simulink model "ASM_Traffic_V2X_Complete_Model_2"  (R2019a)
settings: Solver=ode1  StartTime=SIM.tstart.v  StopTime=Inf  FixedStep=SIM.StepSize.v  RelTol=1e-3
PostLoadFcn:
  | if any(exist('dsrtsu_mdlpostloadfcn', 'file') ~= 0), dsrtsu_mdlpostloadfcn('Execute', bdroot); end
  | try, asm_mdl_postloadfcn(bdroot, 'UpdateModel', 2200); catch, disp(lasterr); end,
undefined symbols (not defined in the file): _SensorPnts_1, _SensorPnts_13, _SensorPnts_17, _SensorPnts_21, _SensorPnts_25, _SensorPnts_29, _SensorPnts_33, _SensorPnts_37, _SensorPnts_41, _SensorPnts_45, _SensorPnts_49, _SensorPnts_5, _SensorPnts_53, _SensorPnts_57, _SensorPnts_9, _to_, CPT, G5A, ITS, MDL, rad, s_to_rpm, SIM
libraries: simulink x169, ASM_VehicleDynamics_lib x126, ASM_Traffic_lib x83, ASM_Utils_lib x49, mdbs x45, ASM_Environment_lib x17, dspindex x12, dsaV2xLibraryAux x10, dsmpblib x6, dsaV2xAsn1Library x4, dsaV2xLibrary x4, ASM_BrakeHydraulics_lib x4
(part 25 of 36)

== system ASM_Traffic_V2X_Complete_Model_2/MDL/Environment/Traffic/Sensors/Object_Sensor_2D/SensorParameters ==
  Demux{,1..6} (7 alike) : Demux  Outputs=3
  Mux{1..7} (7 alike) : Mux  Inputs=14
  OBJECT_SENSOR_2D_PARAMETERS_1 : ASM_Traffic_lib/Sensors/Object_Sensor_2D/OBJECT_SENSOR_2D_PARAMETERS  Tag=ASM_SUBCOMPONENT  Sw_Sensor_Enable=MDL.Traffic.Sensors.ObjectSensor2D_1.Sw_Sensor_Enable  Const_SensorIdx=MDL.Traffic.Sensors.ObjectSensor2D_1.Const_SensorIdx  Const_t_Offs_Sensor=MDL.Traffic.Sensors.ObjectSensor2D_1.Const_t_Offs_Sensor  Const_t_Cycle_Sensor=MDL.Traffic.Sensors.ObjectSensor2D_1.Const_t_Cycle_Sensor  Const_t_Delay_SensorOutput=MDL.Traffic.Sensors.ObjectSensor2D_1.Const_t_Delay_SensorOutput  Const_Pos_Sensor_Apex_CoorSys_V=MDL.Traffic.Sensors.ObjectSensor2D_1.Const_Pos_Sensor_Apex_CoorSys_V  Const_Angle_z_Orientation_Sensor_CoorSys_V=MDL.Traffic.Sensors.ObjectSensor2D_1.Const_Angle_z_Orientation_Sensor_CoorSys_V  Const_Angle_ScopeZone_Horizontal=MDL.Traffic.Sensors.ObjectSensor2D_1.Const_Angle_ScopeZone_Horizontal  Const_Length_ScopeZone=MDL.Traffic.Sensors.ObjectSensor2D_1.Const_Length_ScopeZone  Const_Num_SensorRays_Used=MDL.Traffic.Sensors.ObjectSensor2D_1.Const_Num_SensorRays_Used  Sw_Sensor_Detection_Mode=MDL.Traffic.Sensors.ObjectSensor2D_1.Sw_Sensor_Detection_Mode  Sw_Object_Detection_Mode=MDL.Traffic.Sensors.ObjectSensor2D_1.Sw_Object_Detection_Mode  ASMProperties=struct('Name','OBJECT_SENSOR_2D_PARAMETERS','Version','5.0','Library','ASM_Traffic_lib')  ASMInstanceName=object_sensor_2d_parameters  ASMInstanceID=1
  OBJECT_SENSOR_2D_PARAMETERS_2 : ASM_Traffic_lib/Sensors/Object_Sensor_2D/OBJECT_SENSOR_2D_PARAMETERS  Tag=ASM_SUBCOMPONENT  Sw_Sensor_Enable=MDL.Traffic.Sensors.ObjectSensor2D_2.Sw_Sensor_Enable  Const_SensorIdx=MDL.Traffic.Sensors.ObjectSensor2D_2.Const_SensorIdx  Const_t_Offs_Sensor=MDL.Traffic.Sensors.ObjectSensor2D_2.Const_t_Offs_Sensor  Const_t_Cycle_Sensor=MDL.Traffic.Sensors.ObjectSensor2D_2.Const_t_Cycle_Sensor  Const_t_Delay_SensorOutput=MDL.Traffic.Sensors.ObjectSensor2D_2.Const_t_Delay_SensorOutput  Const_Pos_Sensor_Apex_CoorSys_V=MDL.Traffic.Sensors.ObjectSensor2D_2.Const_Pos_Sensor_Apex_CoorSys_V  Const_Angle_z_Orientation_Sensor_CoorSys_V=MDL.Traffic.Sensors.ObjectSensor2D_2.Const_Angle_z_Orientation_Sensor_CoorSys_V  Const_Angle_ScopeZone_Horizontal=MDL.Traffic.Sensors.ObjectSensor2D_2.Const_Angle_ScopeZone_Horizontal  Const_Length_ScopeZone=MDL.Traffic.Sensors.ObjectSensor2D_2.Const_Length_ScopeZone  Const_Num_SensorRays_Used=MDL.Traffic.Sensors.ObjectSensor2D_2.Const_Num_SensorRays_Used  Sw_Sensor_Detection_Mode=MDL.Traffic.Sensors.ObjectSensor2D_2.Sw_Sensor_Detection_Mode  Sw_Object_Detection_Mode=MDL.Traffic.Sensors.ObjectSensor2D_2.Sw_Object_Detection_Mode  ASMProperties=struct('Name','OBJECT_SENSOR_2D_PARAMETERS','Version','5.0','Library','ASM_Traffic_lib')  ASMInstanceName=object_sensor_2d_parameters  ASMInstanceID=2
      settings: AttributesFormatString=Instance Name: object_sensor_2d_parameters\nInstance ID: 2
  OBJECT_SENSOR_2D_PARAMETERS_3 : ASM_Traffic_lib/Sensors/Object_Sensor_2D/OBJECT_SENSOR_2D_PARAMETERS  Tag=ASM_SUBCOMPONENT  Sw_Sensor_Enable=MDL.Traffic.Sensors.ObjectSensor2D_3.Sw_Sensor_Enable  Const_SensorIdx=MDL.Traffic.Sensors.ObjectSensor2D_3.Const_SensorIdx  Const_t_Offs_Sensor=MDL.Traffic.Sensors.ObjectSensor2D_3.Const_t_Offs_Sensor  Const_t_Cycle_Sensor=MDL.Traffic.Sensors.ObjectSensor2D_3.Const_t_Cycle_Sensor  Const_t_Delay_SensorOutput=MDL.Traffic.Sensors.ObjectSensor2D_3.Const_t_Delay_SensorOutput  Const_Pos_Sensor_Apex_CoorSys_V=MDL.Traffic.Sensors.ObjectSensor2D_3.Const_Pos_Sensor_Apex_CoorSys_V  Const_Angle_z_Orientation_Sensor_CoorSys_V=MDL.Traffic.Sensors.ObjectSensor2D_3.Const_Angle_z_Orientation_Sensor_CoorSys_V  Const_Angle_ScopeZone_Horizontal=MDL.Traffic.Sensors.ObjectSensor2D_3.Const_Angle_ScopeZone_Horizontal  Const_Length_ScopeZone=MDL.Traffic.Sensors.ObjectSensor2D_3.Const_Length_ScopeZone  Const_Num_SensorRays_Used=MDL.Traffic.Sensors.ObjectSensor2D_3.Const_Num_SensorRays_Used  Sw_Sensor_Detection_Mode=MDL.Traffic.Sensors.ObjectSensor2D_3.Sw_Sensor_Detection_Mode  Sw_Object_Detection_Mode=MDL.Traffic.Sensors.ObjectSensor2D_3.Sw_Object_Detection_Mode  ASMProperties=struct('Name','OBJECT_SENSOR_2D_PARAMETERS','Version','5.0','Library','ASM_Traffic_lib')  ASMInstanceName=object_sensor_2d_parameters  ASMInstanceID=3
      settings: AttributesFormatString=Instance Name: object_sensor_2d_parameters\nInstance ID: 3
  OBJECT_SENSOR_2D_PARAMETERS_4 : ASM_Traffic_lib/Sensors/Object_Sensor_2D/OBJECT_SENSOR_2D_PARAMETERS  Tag=ASM_SUBCOMPONENT  Sw_Sensor_Enable=MDL.Traffic.Sensors.ObjectSensor2D_4.Sw_Sensor_Enable  Const_SensorIdx=MDL.Traffic.Sensors.ObjectSensor2D_4.Const_SensorIdx  Const_t_Offs_Sensor=MDL.Traffic.Sensors.ObjectSensor2D_4.Const_t_Offs_Sensor  Const_t_Cycle_Sensor=MDL.Traffic.Sensors.ObjectSensor2D_4.Const_t_Cycle_Sensor  Const_t_Delay_SensorOutput=MDL.Traffic.Sensors.ObjectSensor2D_4.Const_t_Delay_SensorOutput  Const_Pos_Sensor_Apex_CoorSys_V=MDL.Traffic.Sensors.ObjectSensor2D_4.Const_Pos_Sensor_Apex_CoorSys_V  Const_Angle_z_Orientation_Sensor_CoorSys_V=MDL.Traffic.Sensors.ObjectSensor2D_4.Const_Angle_z_Orientation_Sensor_CoorSys_V  Const_Angle_ScopeZone_Horizontal=MDL.Traffic.Sensors.ObjectSensor2D_4.Const_Angle_ScopeZone_Horizontal  Const_Length_ScopeZone=MDL.Traffic.Sensors.ObjectSensor2D_4.Const_Length_ScopeZone  Const_Num_SensorRays_Used=MDL.Traffic.Sensors.ObjectSensor2D_4.Const_Num_SensorRays_Used  Sw_Sensor_Detection_Mode=MDL.Traffic.Sensors.ObjectSensor2D_4.Sw_Sensor_Detection_Mode  Sw_Object_Detection_Mode=MDL.Traffic.Sensors.ObjectSensor2D_4.Sw_Object_Detection_Mode  ASMProperties=struct('Name','OBJECT_SENSOR_2D_PARAMETERS','Version','5.0','Library','ASM_Traffic_lib')  ASMInstanceName=object_sensor_2d_parameters  ASMInstanceID=4
      settings: AttributesFormatString=Instance Name: object_sensor_2d_parameters\nInstance ID: 4
  OBJECT_SENSOR_2D_PARAMETERS_5 : ASM_Traffic_lib/Sensors/Object_Sensor_2D/OBJECT_SENSOR_2D_PARAMETERS  Tag=ASM_SUBCOMPONENT  Sw_Sensor_Enable=MDL.Traffic.Sensors.ObjectSensor2D_5.Sw_Sensor_Enable  Const_SensorIdx=MDL.Traffic.Sensors.ObjectSensor2D_5.Const_SensorIdx  Const_t_Offs_Sensor=MDL.Traffic.Sensors.ObjectSensor2D_5.Const_t_Offs_Sensor  Const_t_Cycle_Sensor=MDL.Traffic.Sensors.ObjectSensor2D_5.Const_t_Cycle_Sensor  Const_t_Delay_SensorOutput=MDL.Traffic.Sensors.ObjectSensor2D_5.Const_t_Delay_SensorOutput  Const_Pos_Sensor_Apex_CoorSys_V=MDL.Traffic.Sensors.ObjectSensor2D_5.Const_Pos_Sensor_Apex_CoorSys_V  Const_Angle_z_Orientation_Sensor_CoorSys_V=MDL.Traffic.Sensors.ObjectSensor2D_5.Const_Angle_z_Orientation_Sensor_CoorSys_V  Const_Angle_ScopeZone_Horizontal=MDL.Traffic.Sensors.ObjectSensor2D_5.Const_Angle_ScopeZone_Horizontal  Const_Length_ScopeZone=MDL.Traffic.Sensors.ObjectSensor2D_5.Const_Length_ScopeZone  Const_Num_SensorRays_Used=MDL.Traffic.Sensors.ObjectSensor2D_5.Const_Num_SensorRays_Used  Sw_Sensor_Detection_Mode=MDL.Traffic.Sensors.ObjectSensor2D_5.Sw_Sensor_Detection_Mode  Sw_Object_Detection_Mode=MDL.Traffic.Sensors.ObjectSensor2D_5.Sw_Object_Detection_Mode  ASMProperties=struct('Name','OBJECT_SENSOR_2D_PARAMETERS','Version','5.0','Library','ASM_Traffic_lib')  ASMInstanceName=object_sensor_2d_parameters  ASMInstanceID=5
      settings: AttributesFormatString=Instance Name: object_sensor_2d_parameters\nInstance ID: 5
  OBJECT_SENSOR_2D_PARAMETERS_6 : ASM_Traffic_lib/Sensors/Object_Sensor_2D/OBJECT_SENSOR_2D_PARAMETERS  Tag=ASM_SUBCOMPONENT  Sw_Sensor_Enable=MDL.Traffic.Sensors.ObjectSensor2D_6.Sw_Sensor_Enable  Const_SensorIdx=MDL.Traffic.Sensors.ObjectSensor2D_6.Const_SensorIdx  Const_t_Offs_Sensor=MDL.Traffic.Sensors.ObjectSensor2D_6.Const_t_Offs_Sensor  Const_t_Cycle_Sensor=MDL.Traffic.Sensors.ObjectSensor2D_6.Const_t_Cycle_Sensor  Const_t_Delay_SensorOutput=MDL.Traffic.Sensors.ObjectSensor2D_6.Const_t_Delay_SensorOutput  Const_Pos_Sensor_Apex_CoorSys_V=MDL.Traffic.Sensors.ObjectSensor2D_6.Const_Pos_Sensor_Apex_CoorSys_V  Const_Angle_z_Orientation_Sensor_CoorSys_V=MDL.Traffic.Sensors.ObjectSensor2D_6.Const_Angle_z_Orientation_Sensor_CoorSys_V  Const_Angle_ScopeZone_Horizontal=MDL.Traffic.Sensors.ObjectSensor2D_6.Const_Angle_ScopeZone_Horizontal  Const_Length_ScopeZone=MDL.Traffic.Sensors.ObjectSensor2D_6.Const_Length_ScopeZone  Const_Num_SensorRays_Used=MDL.Traffic.Sensors.ObjectSensor2D_6.Const_Num_SensorRays_Used  Sw_Sensor_Detection_Mode=MDL.Traffic.Sensors.ObjectSensor2D_6.Sw_Sensor_Detection_Mode  Sw_Object_Detection_Mode=MDL.Traffic.Sensors.ObjectSensor2D_6.Sw_Object_Detection_Mode  ASMProperties=struct('Name','OBJECT_SENSOR_2D_PARAMETERS','Version','5.0','Library','ASM_Traffic_lib')  ASMInstanceName=object_sensor_2d_parameters  ASMInstanceID=6
      settings: AttributesFormatString=Instance Name: object_sensor_2d_parameters\nInstance ID: 6
  OBJECT_SENSOR_2D_PARAMETERS_7 : ASM_Traffic_lib/Sensors/Object_Sensor_2D/OBJECT_SENSOR_2D_PARAMETERS  Tag=ASM_SUBCOMPONENT  Sw_Sensor_Enable=MDL.Traffic.Sensors.ObjectSensor2D_7.Sw_Sensor_Enable  Const_SensorIdx=MDL.Traffic.Sensors.ObjectSensor2D_7.Const_SensorIdx  Const_t_Offs_Sensor=MDL.Traffic.Sensors.ObjectSensor2D_7.Const_t_Offs_Sensor  Const_t_Cycle_Sensor=MDL.Traffic.Sensors.ObjectSensor2D_7.Const_t_Cycle_Sensor  Const_t_Delay_SensorOutput=MDL.Traffic.Sensors.ObjectSensor2D_7.Const_t_Delay_SensorOutput  Const_Pos_Sensor_Apex_CoorSys_V=MDL.Traffic.Sensors.ObjectSensor2D_7.Const_Pos_Sensor_Apex_CoorSys_V  Const_Angle_z_Orientation_Sensor_CoorSys_V=MDL.Traffic.Sensors.ObjectSensor2D_7.Const_Angle_z_Orientation_Sensor_CoorSys_V  Const_Angle_ScopeZone_Horizontal=MDL.Traffic.Sensors.ObjectSensor2D_7.Const_Angle_ScopeZone_Horizontal  Const_Length_ScopeZone=MDL.Traffic.Sensors.ObjectSensor2D_7.Const_Length_ScopeZone  Const_Num_SensorRays_Used=MDL.Traffic.Sensors.ObjectSensor2D_7.Const_Num_SensorRays_Used  Sw_Sensor_Detection_Mode=MDL.Traffic.Sensors.ObjectSensor2D_7.Sw_Sensor_Detection_Mode  Sw_Object_Detection_Mode=MDL.Traffic.Sensors.ObjectSensor2D_7.Sw_Object_Detection_Mode  ASMProperties=struct('Name','OBJECT_SENSOR_2D_PARAMETERS','Version','5.0','Library','ASM_Traffic_lib')  ASMInstanceName=object_sensor_2d_parameters  ASMInstanceID=7
      settings: AttributesFormatString=Instance Name: object_sensor_2d_parameters\nInstance ID: 7
  Vector Concatenate : Concatenate  NumInputs=7  Mode=Multidimensional array  ConcatenateDimension=2
  Sensor_Data[] : Outport
  tag scope: ASMBUS_Environment_Traffic_2DObjSensor1_Parameter=global, ASMBUS_Environment_Traffic_2DObjSensor2_Parameter=global, ASMBUS_Environment_Traffic_2DObjSensor3_Parameter=global, ASMBUS_Environment_Traffic_2DObjSensor4_Parameter=global, ASMBUS_Environment_Traffic_2DObjSensor5_Parameter=global, ASMBUS_Environment_Traffic_2DObjSensor6_Parameter=global, ASMBUS_Environment_Traffic_2DObjSensor7_Parameter=global
  wires:
  OBJECT_SENSOR_2D_PARAMETERS_3/13 -> Mux3/14
  OBJECT_SENSOR_2D_PARAMETERS_4/13 -> Mux4/14
  OBJECT_SENSOR_2D_PARAMETERS_7/13 -> Mux7/14
  OBJECT_SENSOR_2D_PARAMETERS_6/13 -> Mux6/14
  OBJECT_SENSOR_2D_PARAMETERS_5/13 -> Mux5/14
  OBJECT_SENSOR_2D_PARAMETERS_2/13 -> Mux2/14
  OBJECT_SENSOR_2D_PARAMETERS_1/13 -> Mux1/14
  OBJECT_SENSOR_2D_PARAMETERS_7/12 -> Mux7/13
  OBJECT_SENSOR_2D_PARAMETERS_7/11 -> Mux7/12
  OBJECT_SENSOR_2D_PARAMETERS_7/10 -> Mux7/11
  OBJECT_SENSOR_2D_PARAMETERS_7/9 -> Mux7/10
  OBJECT_SENSOR_2D_PARAMETERS_7/8 -> Mux7/9
  OBJECT_SENSOR_2D_PARAMETERS_7/6 -> Mux7/5
  OBJECT_SENSOR_2D_PARAMETERS_7/5 -> Mux7/4
  OBJECT_SENSOR_2D_PARAMETERS_7/4 -> Mux7/3
  OBJECT_SENSOR_2D_PARAMETERS_7/3 -> Mux7/2
  OBJECT_SENSOR_2D_PARAMETERS_7/2 -> Mux7/1
  Demux6/3 -> Mux7/8
  Demux6/2 -> Mux7/7
  Demux6/1 -> Mux7/6
  Mux7/1 -> Vector Concatenate/7
  OBJECT_SENSOR_2D_PARAMETERS_7/7 -> Demux6/1
  OBJECT_SENSOR_2D_PARAMETERS_6/12 -> Mux6/13
  OBJECT_SENSOR_2D_PARAMETERS_6/11 -> Mux6/12
  OBJECT_SENSOR_2D_PARAMETERS_6/10 -> Mux6/11
  OBJECT_SENSOR_2D_PARAMETERS_6/9 -> Mux6/10
  OBJECT_SENSOR_2D_PARAMETERS_6/8 -> Mux6/9
  OBJECT_SENSOR_2D_PARAMETERS_6/6 -> Mux6/5
  OBJECT_SENSOR_2D_PARAMETERS_6/5 -> Mux6/4
  OBJECT_SENSOR_2D_PARAMETERS_6/4 -> Mux6/3
  OBJECT_SENSOR_2D_PARAMETERS_6/3 -> Mux6/2
  OBJECT_SENSOR_2D_PARAMETERS_6/2 -> Mux6/1
  Demux5/3 -> Mux6/8
  Demux5/2 -> Mux6/7
  Demux5/1 -> Mux6/6
  Mux6/1 -> Vector Concatenate/6
  OBJECT_SENSOR_2D_PARAMETERS_6/7 -> Demux5/1
  OBJECT_SENSOR_2D_PARAMETERS_5/12 -> Mux5/13
  OBJECT_SENSOR_2D_PARAMETERS_5/11 -> Mux5/12
  OBJECT_SENSOR_2D_PARAMETERS_5/10 -> Mux5/11
  OBJECT_SENSOR_2D_PARAMETERS_5/9 -> Mux5/10
  OBJECT_SENSOR_2D_PARAMETERS_5/8 -> Mux5/9
  OBJECT_SENSOR_2D_PARAMETERS_5/6 -> Mux5/5
  OBJECT_SENSOR_2D_PARAMETERS_5/5 -> Mux5/4
  OBJECT_SENSOR_2D_PARAMETERS_5/4 -> Mux5/3
  OBJECT_SENSOR_2D_PARAMETERS_5/3 -> Mux5/2
  OBJECT_SENSOR_2D_PARAMETERS_5/2 -> Mux5/1
  Demux4/3 -> Mux5/8
  Demux4/2 -> Mux5/7
  Demux4/1 -> Mux5/6
  Mux5/1 -> Vector Concatenate/5
  OBJECT_SENSOR_2D_PARAMETERS_5/7 -> Demux4/1
  OBJECT_SENSOR_2D_PARAMETERS_4/12 -> Mux4/13
  OBJECT_SENSOR_2D_PARAMETERS_4/11 -> Mux4/12
  OBJECT_SENSOR_2D_PARAMETERS_4/10 -> Mux4/11
  OBJECT_SENSOR_2D_PARAMETERS_4/9 -> Mux4/10
  OBJECT_SENSOR_2D_PARAMETERS_4/8 -> Mux4/9
  OBJECT_SENSOR_2D_PARAMETERS_4/6 -> Mux4/5
  OBJECT_SENSOR_2D_PARAMETERS_4/5 -> Mux4/4
  OBJECT_SENSOR_2D_PARAMETERS_4/4 -> Mux4/3
  OBJECT_SENSOR_2D_PARAMETERS_4/3 -> Mux4/2
  OBJECT_SENSOR_2D_PARAMETERS_4/2 -> Mux4/1
  Demux3/3 -> Mux4/8
  Demux3/2 -> Mux4/7
  Demux3/1 -> Mux4/6
  Mux4/1 -> Vector Concatenate/4
  OBJECT_SENSOR_2D_PARAMETERS_4/7 -> Demux3/1
  OBJECT_SENSOR_2D_PARAMETERS_7/1 -> [ASMBUS_Environment_Traffic_2DObjSensor7_Parameter]
  OBJECT_SENSOR_2D_PARAMETERS_6/1 -> [ASMBUS_Environment_Traffic_2DObjSensor6_Parameter]
  OBJECT_SENSOR_2D_PARAMETERS_5/1 -> [ASMBUS_Environment_Traffic_2DObjSensor5_Parameter]
  OBJECT_SENSOR_2D_PARAMETERS_4/1 -> [ASMBUS_Environment_Traffic_2DObjSensor4_Parameter]
  OBJECT_SENSOR_2D_PARAMETERS_3/12 -> Mux3/13
  OBJECT_SENSOR_2D_PARAMETERS_2/12 -> Mux2/13
  OBJECT_SENSOR_2D_PARAMETERS_1/12 -> Mux1/13
  OBJECT_SENSOR_2D_PARAMETERS_3/11 -> Mux3/12
  OBJECT_SENSOR_2D_PARAMETERS_3/10 -> Mux3/11
  OBJECT_SENSOR_2D_PARAMETERS_3/9 -> Mux3/10
  OBJECT_SENSOR_2D_PARAMETERS_3/8 -> Mux3/9
  OBJECT_SENSOR_2D_PARAMETERS_3/6 -> Mux3/5
  OBJECT_SENSOR_2D_PARAMETERS_3/5 -> Mux3/4
  OBJECT_SENSOR_2D_PARAMETERS_3/4 -> Mux3/3
  OBJECT_SENSOR_2D_PARAMETERS_3/3 -> Mux3/2
  OBJECT_SENSOR_2D_PARAMETERS_3/2 -> Mux3/1
  Demux2/3 -> Mux3/8
  Demux2/2 -> Mux3/7
  Demux2/1 -> Mux3/6
  Mux3/1 -> Vector Concatenate/3
  OBJECT_SENSOR_2D_PARAMETERS_3/7 -> Demux2/1
  OBJECT_SENSOR_2D_PARAMETERS_3/1 -> [ASMBUS_Environment_Traffic_2DObjSensor3_Parameter]
  OBJECT_SENSOR_2D_PARAMETERS_2/11 -> Mux2/12
  OBJECT_SENSOR_2D_PARAMETERS_2/10 -> Mux2/11
  OBJECT_SENSOR_2D_PARAMETERS_2/9 -> Mux2/10
  OBJECT_SENSOR_2D_PARAMETERS_2/8 -> Mux2/9
  OBJECT_SENSOR_2D_PARAMETERS_2/6 -> Mux2/5
  OBJECT_SENSOR_2D_PARAMETERS_2/5 -> Mux2/4
  OBJECT_SENSOR_2D_PARAMETERS_2/4 -> Mux2/3
  OBJECT_SENSOR_2D_PARAMETERS_2/3 -> Mux2/2
  OBJECT_SENSOR_2D_PARAMETERS_2/2 -> Mux2/1
  Demux1/3 -> Mux2/8
  Demux1/2 -> Mux2/7
  Demux1/1 -> Mux2/6
  Mux2/1 -> Vector Concatenate/2
  OBJECT_SENSOR_2D_PARAMETERS_2/7 -> Demux1/1
  OBJECT_SENSOR_2D_PARAMETERS_2/1 -> [ASMBUS_Environment_Traffic_2DObjSensor2_Parameter]
  OBJECT_SENSOR_2D_PARAMETERS_1/11 -> Mux1/12
  OBJECT_SENSOR_2D_PARAMETERS_1/10 -> Mux1/11
  OBJECT_SENSOR_2D_PARAMETERS_1/9 -> Mux1/10
  OBJECT_SENSOR_2D_PARAMETERS_1/8 -> Mux1/9
  OBJECT_SENSOR_2D_PARAMETERS_1/6 -> Mux1/5
  OBJECT_SENSOR_2D_PARAMETERS_1/5 -> Mux1/4
  OBJECT_SENSOR_2D_PARAMETERS_1/4 -> Mux1/3
  OBJECT_SENSOR_2D_PARAMETERS_1/3 -> Mux1/2
  OBJECT_SENSOR_2D_PARAMETERS_1/2 -> Mux1/1
  Demux/3 -> Mux1/8
  Demux/2 -> Mux1/7
  Demux/1 -> Mux1/6
  Vector Concatenate/1 -> Sensor_Data[]/1
  Mux1/1 -> Vector Concatenate/1
  OBJECT_SENSOR_2D_PARAMETERS_1/7 -> Demux/1
  OBJECT_SENSOR_2D_PARAMETERS_1/1 -> [ASMBUS_Environment_Traffic_2DObjSensor1_Parameter]

== system ASM_Traffic_V2X_Complete_Model_2/MDL/Environment/Traffic/Sensors/Object_Sensor_3D/ASMSignalCollector ==
  Bus Creator : BusCreator  Inputs=5
  Bus Creator1 : BusCreator  Inputs=6
  Bus Creator2 : BusCreator  Inputs=6
  Bus Creator3 : BusCreator  Inputs=6
  Bus Selector : BusSelector  OutputSignals=SensorIndex,Info,SensorOutput
  Bus Selector1 : BusSelector  OutputSignals=SensorIndex,Info,SensorOutput
  Bus Selector2 : BusSelector  OutputSignals=SensorIndex,Info,SensorOutput
  tag scope: ASMBUS_Environment_Trafffic_Sensors_Object_Sensor_3D=global
  wires:
  [ASMBUS_Environment_Traffic_3DObjSensor3_RadarEffects] -> Bus Creator3/5  "RadarEffects"
  [ASMBUS_Environment_Traffic_3DObjSensor3_CustomPoints] -> Bus Creator3/6  "CustomPoints"
  [ASMBUS_Environment_Traffic_3DObjSensor2_RadarEffects] -> Bus Creator2/5  "RadarEffects"
  [ASMBUS_Environment_Traffic_3DObjSensor2_CustomPoints] -> Bus Creator2/6  "CustomPoints"
  [ASMBUS_Environment_Traffic_3DObjSensor1_CustomPoints] -> Bus Creator1/6  "CustomPoints"
  [ASMBUS_Environment_Traffic_3DObjSensor1_RadarEffects] -> Bus Creator1/5  "RadarEffects"
  [ASMBUS_Environment_Traffic_SamplePulse] -> Bus Creator/1  "Sample_Pulse"
  [ASMBUS_Environment_Traffic_SensorScheduler] -> Bus Creator/2  "Sensor_Scheduler"
  Bus Selector/3 -> Bus Creator1/4  "<SensorOutput>"
  Bus Selector/2 -> Bus Creator1/3  "<Info>"
  Bus Selector2/3 -> Bus Creator3/4  "<SensorOutput>"
  Bus Selector2/2 -> Bus Creator3/3  "<Info>"
  Bus Selector1/3 -> Bus Creator2/4  "<SensorOutput>"
  Bus Selector1/2 -> Bus Creator2/3  "<Info>"
  Bus Selector1/1 -> Bus Creator2/2  "<SensorIndex>"
  Bus Selector/1 -> Bus Creator1/2  "<SensorIndex>"
  [ASMBUS_Environment_Traffic_3DObjSensor3_Parameters] -> Bus Creator3/1  "Parameter"
  [ASMBUS_Environment_Traffic_3DObjSensor2_Parameters] -> Bus Creator2/1  "Parameter"
  [ASMBUS_Environment_Traffic_3DObjSensor1_Parameters] -> Bus Creator1/1  "Parameter"
  Bus Selector2/1 -> Bus Creator3/2  "<SensorIndex>"
  Bus Creator3/1 -> Bus Creator/5  "Sensor_3_Rear"
  Bus Creator2/1 -> Bus Creator/4  "Sensor_2_Front_Mid"
  Bus Creator1/1 -> Bus Creator/3  "Sensor_1_Front_Long"
  [ASMBUS_Environment_Traffic_3DObjSensor3_SensorSignals] -> Bus Selector2/1
  [ASMBUS_Environment_Traffic_3DObjSensor2_SensorSignals] -> Bus Selector1/1
  [ASMBUS_Environment_Traffic_3DObjSensor1_SensorSignals] -> Bus Selector/1
  Bus Creator/1 -> [ASMBUS_Environment_Trafffic_Sensors_Object_Sensor_3D]  "Object_Sensor_3D"

== system ASM_Traffic_V2X_Complete_Model_2/MDL/Environment/Traffic/Sensors/Object_Sensor_3D/CustomPoints ==
  Enable[0Off|1On] : Inport
  SensorMapping_Data[] : Inport  Port=2
  SensorData[] : Inport  Port=3
  Demux : Demux  Outputs=3
  Sensor1 : Subsystem
  Sensor2 : Subsystem
  Sensor3 : Subsystem
  tag scope: ASMBUS_Environment_Traffic_3DObjSensor1_CustomPoints=global, ASMBUS_Environment_Traffic_3DObjSensor2_CustomPoints=global, ASMBUS_Environment_Traffic_3DObjSensor3_CustomPoints=global
  wires:
  Sensor3/1(CustomPoints_Signals[]) -> [ASMBUS_Environment_Traffic_3DObjSensor3_CustomPoints]
  Sensor2/1(CustomPoints_Signals[]) -> [ASMBUS_Environment_Traffic_3DObjSensor2_CustomPoints]
  Sensor1/1(CustomPoints_Signals[]) -> [ASMBUS_Environment_Traffic_3DObjSensor1_CustomPoints]
  Enable[0Off|1On]/1 -> Sensor1/1(Enable[0|1]), Sensor2/1(Enable[0|1]), Sensor3/1(Enable[0|1])
  SensorData[]/1 -> Sensor1/3(SensorData[]), Sensor2/3(SensorData[]), Sensor3/3(SensorData[])
  Demux/3 -> Sensor3/2(SensorMapping_Data[])
  Demux/2 -> Sensor2/2(SensorMapping_Data[])
  Demux/1 -> Sensor1/2(SensorMapping_Data[])
  SensorMapping_Data[]/1 -> Demux/1

== system ASM_Traffic_V2X_Complete_Model_2/MDL/Environment/Traffic/Sensors/Object_Sensor_3D/Enable_Object_Sensor_3D ==
  Enable_In[0Off|1On] : Inport
  Constant : Constant  Value=0.5  SampleTime=-1
  Constant1 : Constant  SampleTime=-1
  Constant2 : Constant  Value=0  SampleTime=-1
  Enable_Sensor : Gain
  Multiport Switch : MultiPortSwitch  DataPortOrder=Zero-based contiguous  Inputs=2  zeroidx=on
  Relational Operator : RelationalOperator  Operator=>  OutDataTypeStr=boolean  RndMeth=Nearest
  Enable_Out[0Off|1On] : Outport
  wires:
  Constant2/1 -> Multiport Switch/2
  Constant1/1 -> Multiport Switch/3
  Constant/1 -> Relational Operator/2
  Multiport Switch/1 -> Enable_Out[0Off|1On]/1
  Relational Operator/1 -> Multiport Switch/1
  Enable_Sensor/1 -> Relational Operator/1
  Enable_In[0Off|1On]/1 -> Enable_Sensor/1

== system ASM_Traffic_V2X_Complete_Model_2/MDL/Environment/Traffic/Sensors/Object_Sensor_3D/RadarEffects ==
  Enable[0Off|1On] : Inport
  SensorMapping_Data[] : Inport  Port=2
  SensorData[] : Inport  Port=3
  Angle_Vehicle_CoorSys_E[x;y;z][deg] : Inport  Port=4
  Pos_Vehicle_CoorSys_E[x;y;z][m] : Inport  Port=5
  Demux1 : Demux  Outputs=3
  Sensor1 : Subsystem
  Sensor2 : Subsystem
  Sensor3 : Subsystem
  tag scope: ASMBUS_Environment_Traffic_3DObjSensor1_RadarEffects=global, ASMBUS_Environment_Traffic_3DObjSensor2_RadarEffects=global, ASMBUS_Environment_Traffic_3DObjSensor3_RadarEffects=global
  wires:
  Sensor3/1(RadarEffect_Signals[]) -> [ASMBUS_Environment_Traffic_3DObjSensor3_RadarEffects]
  Demux1/3 -> Sensor3/2(SensorMapping_Data[])
  Demux1/2 -> Sensor2/2(SensorMapping_Data[])
  Sensor2/1(RadarEffect_Signals[]) -> [ASMBUS_Environment_Traffic_3DObjSensor2_RadarEffects]
  Sensor1/1(RadarEffect_Signals[]) -> [ASMBUS_Environment_Traffic_3DObjSensor1_RadarEffects]
  Pos_Vehicle_CoorSys_E[x;y;z][m]/1 -> Sensor3/5(Pos_Vehicle_CoorSys_E[x;y;z][m]), Sensor2/5(Pos_Vehicle_CoorSys_E[x;y;z][m]), Sensor1/5(Pos_Vehicle_CoorSys_E[x;y;z][m])
  Angle_Vehicle_CoorSys_E[x;y;z][deg]/1 -> Sensor2/4(Angle_Vehicle_CoorSys_E[x;y;z][deg]), Sensor3/4(Angle_Vehicle_CoorSys_E[x;y;z][deg]), Sensor1/4(Angle_Vehicle_CoorSys_E[x;y;z][deg])
  Demux1/1 -> Sensor1/2(SensorMapping_Data[])
  SensorMapping_Data[]/1 -> Demux1/1
  SensorData[]/1 -> Sensor2/3(Sensor_Data[]), Sensor3/3(Sensor_Data[]), Sensor1/3(Sensor_Data[])
  Enable[0Off|1On]/1 -> Sensor1/1(Enable[0|1]), Sensor2/1(Enable[0|1]), Sensor3/1(Enable[0|1])

== system ASM_Traffic_V2X_Complete_Model_2/MDL/Environment/Traffic/Sensors/Object_Sensor_3D/ScheduleAndCalculateSensor ==
  Sensor_Data[] : Inport
  Enable[0Off|1On] : Inport  Port=2
  Fellows_Signals : Inport  Port=3
  VehicleDynamics_Signals : Inport  Port=4
  Objects_Signals : Inport  Port=5
  Road_Signals : Inport  Port=6
  Bus Selector : BusSelector  OutputSignals=VehicleMovement.Positions.Angle_Vehicle_CoorSys_E[x;y;z][deg].Angle_Vehicle_CoorSys_E[x;y;z][deg],VehicleMovement.Positions.Pos_Vehicle_CoorSys_E[x;y;z][m].Pos_Vehicle_CoorSys_E[x;y;z][m]
  Bus Selector2 : BusSelector  OutputSignals=Angle_Fellows[x;y;z][deg],Pos_Fellows_MainPnt_CoorSys_E[x;y;z][m],Flag_FellowUsed[0|1]
  Bus Selector3 : BusSelector  OutputSignals=FellowsGeometry.PosVec_MainPnt_Fellows[x;y;z][m],FellowsGeometry.Size_Fellows[m],TrafficObject_Type_Data[],TrafficObject_Type_Fellows[]
  Bus Selector4 : BusSelector  OutputSignals=TrafficObject_Data[]  OutputAsBus=on
  Bus to Vector : BusToVector
  Mux : Mux  Inputs=2
  OBJECT_SENSOR_3D_CALCULATION : ASM_Traffic_lib/Sensors/Object_Sensor_3D/OBJECT_SENSOR_3D_CALCULATION  Tag=ASM_SUBCOMPONENT  Const_Sensor_Output_Dimension=MDL.Traffic.Sensors.ObjectSensor3D_Calculation.Const_Sensor_Output_Dimension  Sw_Enable_Static_Objects=MDL.Traffic.Sensors.ObjectSensor3D_Calculation.Sw_Enable_Static_Objects  Sw_Output_Mode=MDL.Traffic.Sensors.ObjectSensor3D_Calculation.Sw_Output_Mode  ASMProperties=struct('Name','OBJECT_SENSOR_3D_CALCULATION','Version','7.0','Library','ASM_Traffic_lib')  ASMInstanceName=object_sensor_3d_calculation  ASMInstanceID=1
  OBJECT_SENSOR_3D_PARAM_SELECTION : ASM_Traffic_lib/Sensors/Object_Sensor_3D/OBJECT_SENSOR_3D_PARAM_SELECTION  ASMProperties=struct('Name','OBJECT_SENSOR_3D_PARAM_SELECTION','Version','4.0','Library','ASM_Traffic_lib')  ASMInstanceName=object_sensor_3d_param_selection  ASMInstanceID=1
  OBJECT_SENSOR_3D_PARAM_VECTORIZATION : ASM_Traffic_lib/Sensors/Object_Sensor_3D/OBJECT_SENSOR_3D_PARAM_VECTORIZATION  ASMProperties=struct('Name','OBJECT_SENSOR_3D_PARAM_VECTORIZATION','Version','4.0','Library','ASM_Traffic_lib')  ASMInstanceName=object_sensor_3d_param_vectorization  ASMInstanceID=1
  Reshape2 : Reshape
  SAMPLE_PULSE : ASM_Traffic_lib/Sensors/Scheduling/SAMPLE_PULSE  Tag=ASM_SUBCOMPONENT  Sw_SamplePulse=MDL.Traffic.Sensors.SamplePulse.Sw_SamplePulse  Const_t_Offs_Pulse=MDL.Traffic.Sensors.SamplePulse.Const_t_Offs_Pulse  Const_t_Cycle_Pulse=MDL.Traffic.Sensors.SamplePulse.Const_t_Cycle_Pulse  StepSize=SIM.StepSize  ASMProperties=struct('Name','SAMPLE_PULSE','Version','3.0','Library','ASM_Traffic_lib')  ASMInstanceName=sample_pulse  ASMInstanceID=1
  SENSOR_SCHEDULER : ASM_Traffic_lib/Sensors/Scheduling/SENSOR_SCHEDULER  StepSize=SIM.StepSize  ASMProperties=struct('Name','SENSOR_SCHEDULER','Version','4.0','Library','ASM_Traffic_lib')  ASMInstanceName=sensor_scheduler  ASMInstanceID=1
  SampleAndHold : Subsystem  TreatAsAtomicUnit=on
  Terminator{1..4,7} (5 alike) : Terminator
  SensorMapping_Data[] : Outport
  SensorSignals : Outport  Port=2
  SensorData[] : Outport  Port=3
  Angle_Vehicle_CoorSys_E_Sampled[x,y;z][deg] : Outport  Port=4
  Pos_Vehicle_CoorSys_E_Sampled[x,y;z][m] : Outport  Port=5
  tag scope: ASMBUS_Environment_Traffic_SamplePulse=global, ASMBUS_Environment_Traffic_SensorScheduler=global
  wires:
  OBJECT_SENSOR_3D_CALCULATION/3 -> SensorData[]/1
  Bus Selector4/1 -> OBJECT_SENSOR_3D_CALCULATION/13
  SENSOR_SCHEDULER/4 -> Mux/2
  Mux/1 -> OBJECT_SENSOR_3D_CALCULATION/1
  SENSOR_SCHEDULER/3 -> Terminator7/1
  SampleAndHold/4(Out4) -> OBJECT_SENSOR_3D_CALCULATION/7
  SampleAndHold/3(Out3) -> OBJECT_SENSOR_3D_CALCULATION/6
  SampleAndHold/5(Out5) -> OBJECT_SENSOR_3D_CALCULATION/8
  SampleAndHold/2(Out2) -> OBJECT_SENSOR_3D_CALCULATION/5, Pos_Vehicle_CoorSys_E_Sampled[x,y;z][m]/1
  SampleAndHold/1(Out1) -> OBJECT_SENSOR_3D_CALCULATION/4, Angle_Vehicle_CoorSys_E_Sampled[x,y;z][deg]/1
  SENSOR_SCHEDULER/9 -> Terminator4/1
  SENSOR_SCHEDULER/5 -> OBJECT_SENSOR_3D_CALCULATION/2
  Bus Selector2/3 -> SampleAndHold/5(In5)  "<Flag_FellowUsed[0|1]>"
  SENSOR_SCHEDULER/2 -> SensorMapping_Data[]/1
  SENSOR_SCHEDULER/6 -> OBJECT_SENSOR_3D_PARAM_SELECTION/1
  Bus to Vector/1 -> OBJECT_SENSOR_3D_CALCULATION/10
  Fellows_Signals/1 -> Bus Selector2/1
  VehicleDynamics_Signals/1 -> Bus Selector/1
  Road_Signals/1 -> Bus Selector4/1
  Bus Selector3/3 -> OBJECT_SENSOR_3D_CALCULATION/11  "<TrafficObject_Type_Data[]>"
  Bus Selector/2 -> SampleAndHold/2(In2)  "<Pos_Vehicle_CoorSys_E[x;y;z][m]>"
  Bus Selector/1 -> SampleAndHold/1(In1)  "<Angle_Vehicle_CoorSys_E[x;y;z][deg]>"
  Bus Selector2/2 -> SampleAndHold/4(In4)  "<Pos_Fellows_MainPnt_CoorSys_E[x;y;z][m]>"
  Bus Selector3/1 -> Reshape2/1  "<PosVec_MainPnt_Fellows[x;y;z][m]>"
  Bus Selector3/4 -> OBJECT_SENSOR_3D_CALCULATION/12  "<TrafficObject_Type_Fellows[]>"
  Bus Selector3/2 -> Bus to Vector/1  "<Size_Fellows[m]>"
  Objects_Signals/1 -> Bus Selector3/1
  Bus Selector2/1 -> SampleAndHold/3(In3)  "<Angle_Fellows[x;y;z][deg]>"
  Reshape2/1 -> OBJECT_SENSOR_3D_CALCULATION/9
  Sensor_Data[]/1 -> OBJECT_SENSOR_3D_PARAM_VECTORIZATION/1
  Enable[0Off|1On]/1 -> SAMPLE_PULSE/1, Mux/1, SENSOR_SCHEDULER/1
  SENSOR_SCHEDULER/7 -> Terminator2/1
  OBJECT_SENSOR_3D_CALCULATION/1 -> Terminator3/1
  OBJECT_SENSOR_3D_PARAM_SELECTION/1 -> OBJECT_SENSOR_3D_CALCULATION/3
  SENSOR_SCHEDULER/8 -> Terminator1/1
  OBJECT_SENSOR_3D_CALCULATION/2 -> SensorSignals/1
  SENSOR_SCHEDULER/1 -> [ASMBUS_Environment_Traffic_SensorScheduler]
  OBJECT_SENSOR_3D_PARAM_VECTORIZATION/1 -> SENSOR_SCHEDULER/2
  OBJECT_SENSOR_3D_PARAM_VECTORIZATION/2 -> OBJECT_SENSOR_3D_PARAM_SELECTION/2
  SAMPLE_PULSE/2 -> SampleAndHold/Enable
  SAMPLE_PULSE/1 -> [ASMBUS_Environment_Traffic_SamplePulse]

== system ASM_Traffic_V2X_Complete_Model_2/MDL/Environment/Traffic/Sensors/Object_Sensor_3D/SensorMapping ==
  Enable[0Off|1On] : Inport
  SensorMapping_Data[] : Inport  Port=2
  SensorSignals : Inport  Port=3
  Demux : Demux  Outputs=3
  NearestSurfaceMapping : Subsystem
  OBJECT_SENSOR_3D_MAPPING1 : ASM_Traffic_lib/Sensors/Object_Sensor_3D/OBJECT_SENSOR_3D_MAPPING  ASMProperties=struct('Name','OBJECT_SENSOR_3D_MAPPING','Version','8.0','Library','ASM_Traffic_lib')  ASMInstanceName=object_sensor_3d_mapping  ASMInstanceID=1
  OBJECT_SENSOR_3D_MAPPING2 : ASM_Traffic_lib/Sensors/Object_Sensor_3D/OBJECT_SENSOR_3D_MAPPING  ASMProperties=struct('Name','OBJECT_SENSOR_3D_MAPPING','Version','8.0','Library','ASM_Traffic_lib')  ASMInstanceName=object_sensor_3d_mapping  ASMInstanceID=1
  OBJECT_SENSOR_3D_MAPPING3 : ASM_Traffic_lib/Sensors/Object_Sensor_3D/OBJECT_SENSOR_3D_MAPPING  ASMProperties=struct('Name','OBJECT_SENSOR_3D_MAPPING','Version','8.0','Library','ASM_Traffic_lib')  ASMInstanceName=object_sensor_3d_mapping  ASMInstanceID=1
  Signals_to_ACC_SoftECU : Subsystem
  Sensor_Signals : Outport
  tag scope: ASMBUS_Environment_Traffic_3DObjSensor1_SensorSignals=global, ASMBUS_Environment_Traffic_3DObjSensor2_SensorSignals=global, ASMBUS_Environment_Traffic_3DObjSensor3_SensorSignals=global
  wires:
  Enable[0Off|1On]/1 -> OBJECT_SENSOR_3D_MAPPING2/1, OBJECT_SENSOR_3D_MAPPING3/1, OBJECT_SENSOR_3D_MAPPING1/1
  Demux/2 -> OBJECT_SENSOR_3D_MAPPING2/2
  OBJECT_SENSOR_3D_MAPPING3/1 -> NearestSurfaceMapping/3(Sensor3_Signals[]), [ASMBUS_Environment_Traffic_3DObjSensor3_SensorSignals]
  OBJECT_SENSOR_3D_MAPPING2/1 -> Signals_to_ACC_SoftECU/2(Sensor_2_ACC_In), NearestSurfaceMapping/2(Sensor2_Signals[]), [ASMBUS_Environment_Traffic_3DObjSensor2_SensorSignals]
  SensorSignals/1 -> OBJECT_SENSOR_3D_MAPPING2/3, OBJECT_SENSOR_3D_MAPPING3/3, OBJECT_SENSOR_3D_MAPPING1/3
  SensorMapping_Data[]/1 -> Demux/1
  Signals_to_ACC_SoftECU/1(Sensor_Signals) -> Sensor_Signals/1
  OBJECT_SENSOR_3D_MAPPING1/1 -> Signals_to_ACC_SoftECU/1(Sensor_1_ACC_In), [ASMBUS_Environment_Traffic_3DObjSensor1_SensorSignals], NearestSurfaceMapping/1(Sensor1_Signals[])
  Demux/3 -> OBJECT_SENSOR_3D_MAPPING3/2
  Demux/1 -> OBJECT_SENSOR_3D_MAPPING1/2

== system ASM_Traffic_V2X_Complete_Model_2/MDL/Environment/Traffic/Sensors/Object_Sensor_3D/SensorParameters ==
  ObjectSensor3DParameters_1 : Subsystem
  ObjectSensor3DParameters_2 : Subsystem
  ObjectSensor3DParameters_3 : Subsystem
  Vector Concatenate : Concatenate  NumInputs=3  Mode=Multidimensional array  ConcatenateDimension=2
  Sensor_Data[] : Outport
  wires:
  ObjectSensor3DParameters_3/1(Sensor_Parameters[]) -> Vector Concatenate/3
  ObjectSensor3DParameters_2/1(Sensor_Parameters[]) -> Vector Concatenate/2
  ObjectSensor3DParameters_1/1(Sensor_Parameters[]) -> Vector Concatenate/1
  Vector Concatenate/1 -> Sensor_Data[]/1

== system ASM_Traffic_V2X_Complete_Model_2/MDL/Environment/Traffic/Sensors/Sensors_Common_Signals/Delay ==
  Enable_Sensor_Scheduling_In[0Off|1On] : Inport
  Unit Delay{,1..29} (30 alike) : UnitDelay  SampleTime=-1
  Enable_Sensor_Scheduling_Out[0Off|1On] : Outport
  wires:
  Unit Delay29/1 -> Enable_Sensor_Scheduling_Out[0Off|1On]/1
  Unit Delay19/1 -> Unit Delay20/1
  Unit Delay28/1 -> Unit Delay29/1
  Unit Delay27/1 -> Unit Delay28/1
  Unit Delay26/1 -> Unit Delay27/1
  Unit Delay25/1 -> Unit Delay26/1
  Unit Delay24/1 -> Unit Delay25/1
  Unit Delay23/1 -> Unit Delay24/1
  Unit Delay22/1 -> Unit Delay23/1
  Unit Delay21/1 -> Unit Delay22/1
  Unit Delay20/1 -> Unit Delay21/1
  Unit Delay10/1 -> Unit Delay11/1
  Unit Delay11/1 -> Unit Delay12/1
  Unit Delay12/1 -> Unit Delay13/1
  Unit Delay13/1 -> Unit Delay14/1
  Unit Delay14/1 -> Unit Delay15/1
  Unit Delay15/1 -> Unit Delay16/1
  Unit Delay16/1 -> Unit Delay17/1
  Unit Delay17/1 -> Unit Delay18/1
  Unit Delay18/1 -> Unit Delay19/1
  Unit Delay9/1 -> Unit Delay10/1
  Unit Delay8/1 -> Unit Delay9/1
  Unit Delay7/1 -> Unit Delay8/1
  Unit Delay6/1 -> Unit Delay7/1
  Unit Delay5/1 -> Unit Delay6/1
  Unit Delay4/1 -> Unit Delay5/1
  Unit Delay3/1 -> Unit Delay4/1
  Unit Delay2/1 -> Unit Delay3/1
  Unit Delay1/1 -> Unit Delay2/1
  Unit Delay/1 -> Unit Delay1/1
  Enable_Sensor_Scheduling_In[0Off|1On]/1 -> Unit Delay/1

== system ASM_Traffic_V2X_Complete_Model_2/MDL/Environment/Traffic/Sensors/Sensors_Common_Signals/SignalCollector ==
  Enable_SensorScheduling[0Off|1On] : Inport
  Bus Creator2 : BusCreator  Inputs=1
  ASMSignalBus : Outport
  wires:
  Enable_SensorScheduling[0Off|1On]/1 -> Bus Creator2/1  "Enable_SensorScheduling[0Off|1On]"
  Bus Creator2/1 -> ASMSignalBus/1  "Sensors_Common"

== system ASM_Traffic_V2X_Complete_Model_2/MDL/Environment/Traffic/Sensors/Traffic_Sign_Sensor/ASMSignalCollector ==
  Bus Creator1 : BusCreator  Inputs=3
  Bus Creator2 : BusCreator  Inputs=1
  Bus Selector : BusSelector  OutputSignals=Info,SensorOutput[]
  tag scope: ASMBUS_Environment_Traffic_Sensors_Traffic_Sign_Sensor_dyn=global
  wires:
  Bus Creator2/1 -> [ASMBUS_Environment_Traffic_Sensors_Traffic_Sign_Sensor_dyn]  "TrafficSign_Sensor_Dyn"
  Bus Creator1/1 -> Bus Creator2/1  "Sensor_Front_1"
  Bus Selector/2 -> Bus Creator1/2  "<SensorOutput[]>"
  Bus Selector/1 -> Bus Creator1/1  "<Info>"
  [ASMBUS_Traf_Sensors_Traffic_Sign_Sensor_dyn_1_Parameters] -> Bus Creator1/3  "Parameters"
  [ASMBUS_Traf_Sensors_dyn_Traffic_Sign_Sensor_1] -> Bus Selector/1

== system ASM_Traffic_V2X_Complete_Model_2/MDL/Environment/Traffic/Sensors/Traffic_Sign_Sensor/Enable_Traffic_Sign_Sensor ==
  Enable_In[0Off|1On] : Inport
  Constant : Constant  Value=0.5  SampleTime=-1
  Constant1 : Constant  SampleTime=-1
  Constant2 : Constant  Value=0  SampleTime=-1
  Enable_Sensor : Gain
  Multiport Switch : MultiPortSwitch  DataPortOrder=Zero-based contiguous  Inputs=2  zeroidx=on
  Relational Operator : RelationalOperator  Operator=>  OutDataTypeStr=boolean  RndMeth=Nearest
  Enable_Out[0Off|1On] : Outport
  wires:
  Constant2/1 -> Multiport Switch/2
  Constant1/1 -> Multiport Switch/3
  Constant/1 -> Relational Operator/2
  Multiport Switch/1 -> Enable_Out[0Off|1On]/1
  Relational Operator/1 -> Multiport Switch/1
  Enable_Sensor/1 -> Relational Operator/1
  Enable_In[0Off|1On]/1 -> Enable_Sensor/1

== system ASM_Traffic_V2X_Complete_Model_2/MDL/Environment/Traffic/Sensors/Traffic_Sign_Sensor/Objects_DataStreams ==
  Bus Selector : BusSelector  OutputSignals=Objects_DataStreams[].DataStream_1[].DataStream_1[],Objects_DataStreams[].DataStream_2[].DataStream_2[],Objects_DataStreams[].DataStream_3[].DataStream_3[],Objects_DataStreams[].DataStream_4[].DataStream_4[],Objects_DataStreams[].DataStream_5[].DataStream_5[],Objects_DataStreams[].DataStream_6[].DataStream_6[],Objects_DataStreams[].DataStream_7[].DataStream_7[],Objects_DataStreams[].DataStream_8[].DataStream_8[]
  Mux : Mux  Inputs=8
  TrafficObjects_States[] : Outport
  wires:
  Bus Selector/8 -> Mux/8  "<DataStream_8[]>"
  Bus Selector/7 -> Mux/7  "<DataStream_7[]>"
  Bus Selector/6 -> Mux/6  "<DataStream_6[]>"
  Bus Selector/5 -> Mux/5  "<DataStream_5[]>"
  Bus Selector/4 -> Mux/4  "<DataStream_4[]>"
  Bus Selector/3 -> Mux/3  "<DataStream_3[]>"
  Bus Selector/2 -> Mux/2  "<DataStream_2[]>"
  Bus Selector/1 -> Mux/1  "<DataStream_1[]>"
  Mux/1 -> TrafficObjects_States[]/1
  [TAG_Objects_DataStreams] -> Bus Selector/1

== system ASM_Traffic_V2X_Complete_Model_2/MDL/SoftECU/Soft_ECU_ACC/Map_Inputs/Maneuver/pos_edge_detection ==
  In1 : Inport
  Memory : Memory
  Relational Operator : RelationalOperator  Operator=>  OutDataTypeStr=boolean  RndMeth=Nearest
  Out1 : Outport
  wires:
  Memory/1 -> Relational Operator/2
  Relational Operator/1 -> Out1/1
  In1/1 -> Memory/1, Relational Operator/1

== system ASM_Traffic_V2X_Complete_Model_2/MDL/SoftECU/Soft_ECU_ACC/Map_Inputs/Maneuver/pos_edge_detection1 ==
  In1 : Inport
  Memory : Memory
  Relational Operator : RelationalOperator  Operator=>  OutDataTypeStr=boolean  RndMeth=Nearest
  Out1 : Outport
  wires:
  In1/1 -> Relational Operator/1, Memory/1
  Relational Operator/1 -> Out1/1
  Memory/1 -> Relational Operator/2

== system ASM_Traffic_V2X_Complete_Model_2/MDL/SoftECU/Soft_ECU_ACC/Map_Inputs/Maneuver/pos_edge_detection2 ==
  In1 : Inport
  Memory : Memory
  Relational Operator : RelationalOperator  Operator=>  OutDataTypeStr=boolean  RndMeth=Nearest
  Out1 : Outport
  wires:
  Memory/1 -> Relational Operator/2
  Relational Operator/1 -> Out1/1
  In1/1 -> Memory/1, Relational Operator/1

== system ASM_Traffic_V2X_Complete_Model_2/MDL/SoftECU/Soft_ECU_ACC/Map_Inputs/Maneuver/pos_edge_detection3 ==
  In1 : Inport
  Memory : Memory
  Relational Operator : RelationalOperator  Operator=>  OutDataTypeStr=boolean  RndMeth=Nearest
  Out1 : Outport
  wires:
  In1/1 -> Relational Operator/1, Memory/1
  Relational Operator/1 -> Out1/1
  Memory/1 -> Relational Operator/2

== system ASM_Traffic_V2X_Complete_Model_2/MDLUserInterface/Environment/MDL_DISP/Traffic/Custom_Sensor/Angle_Hor_Rel[deg] ==
  In1 : Inport
  Out1 : Outport
  wires:
  In1/1 -> Out1/1

== system ASM_Traffic_V2X_Complete_Model_2/MDLUserInterface/Environment/MDL_DISP/Traffic/Custom_Sensor/Angle_Hor_Rel[deg]1 ==
  In1 : Inport
  Out1 : Outport
  wires:
  In1/1 -> Out1/1

== system ASM_Traffic_V2X_Complete_Model_2/MDLUserInterface/Environment/MDL_DISP/Traffic/Custom_Sensor/Angle_Ver_Rel[deg] ==
  In1 : Inport
  Out1 : Outport
  wires:
  In1/1 -> Out1/1

== system ASM_Traffic_V2X_Complete_Model_2/MDLUserInterface/Environment/MDL_DISP/Traffic/Custom_Sensor/Angle_Ver_Rel[deg]1 ==
  In1 : Inport
  Out1 : Outport
  wires:
  In1/1 -> Out1/1

== system ASM_Traffic_V2X_Complete_Model_2/MDLUserInterface/Environment/MDL_DISP/Traffic/Custom_Sensor/CustomSensor_Data_Valid[0|1] ==
  In1 : Inport
  Out1 : Outport
  wires:
  In1/1 -> Out1/1

== system ASM_Traffic_V2X_Complete_Model_2/MDLUserInterface/Environment/MDL_DISP/Traffic/Custom_Sensor/CustomSensor_OutputSfcn_State[] ==
  In1 : Inport
  Out1 : Outport
  wires:
  In1/1 -> Out1/1

== system ASM_Traffic_V2X_Complete_Model_2/MDLUserInterface/Environment/MDL_DISP/Traffic/Custom_Sensor/CustomSensor_ScopezoneSfcn_State[] ==
  In1 : Inport
  Out1 : Outport
  wires:
  In1/1 -> Out1/1

== system ASM_Traffic_V2X_Complete_Model_2/MDLUserInterface/Environment/MDL_DISP/Traffic/Custom_Sensor/CustomValues[] ==
  In1 : Inport
  Out1 : Outport
  wires:
  In1/1 -> Out1/1

== system ASM_Traffic_V2X_Complete_Model_2/MDLUserInterface/Environment/MDL_DISP/Traffic/Custom_Sensor/CustomValues[]1 ==
  In1 : Inport
  Out1 : Outport
  wires:
  In1/1 -> Out1/1

== system ASM_Traffic_V2X_Complete_Model_2/MDLUserInterface/Environment/MDL_DISP/Traffic/Custom_Sensor/Distance[m] ==
  In1 : Inport
  Out1 : Outport
  wires:
  In1/1 -> Out1/1

== system ASM_Traffic_V2X_Complete_Model_2/MDLUserInterface/Environment/MDL_DISP/Traffic/Custom_Sensor/Distance[m]1 ==
  In1 : Inport
  Out1 : Outport
  wires:
  In1/1 -> Out1/1

== system ASM_Traffic_V2X_Complete_Model_2/MDLUserInterface/Environment/MDL_DISP/Traffic/Custom_Sensor/Object_ID[] ==
  In1 : Inport
  Out1 : Outport
  wires:
  In1/1 -> Out1/1

== system ASM_Traffic_V2X_Complete_Model_2/MDLUserInterface/Environment/MDL_DISP/Traffic/Custom_Sensor/Object_ID[]1 ==
  In1 : Inport
  Out1 : Outport
  wires:
  In1/1 -> Out1/1

== system ASM_Traffic_V2X_Complete_Model_2/MDLUserInterface/Environment/MDL_DISP/Traffic/Custom_Sensor/Object_Type[] ==
  In1 : Inport
  Out1 : Outport
  wires:
  In1/1 -> Out1/1

== system ASM_Traffic_V2X_Complete_Model_2/MDLUserInterface/Environment/MDL_DISP/Traffic/Custom_Sensor/Object_Type[]1 ==
  In1 : Inport
  Out1 : Outport
  wires:
  In1/1 -> Out1/1

== system ASM_Traffic_V2X_Complete_Model_2/MDLUserInterface/Environment/MDL_DISP/Traffic/Custom_Sensor/Object_Valid[0|1] ==
  In1 : Inport
  Out1 : Outport
  wires:
  In1/1 -> Out1/1

== system ASM_Traffic_V2X_Complete_Model_2/MDLUserInterface/Environment/MDL_DISP/Traffic/Custom_Sensor/Object_Valid[0|1]1 ==
  In1 : Inport
  Out1 : Outport
  wires:
  In1/1 -> Out1/1

== system ASM_Traffic_V2X_Complete_Model_2/MDLUserInterface/Environment/MDL_DISP/Traffic/Fellow_Movement/CurrentSegment[] ==
  In1 : Inport
  Out1 : Outport
  wires:
  In1/1 -> Out1/1

== system ASM_Traffic_V2X_Complete_Model_2/MDLUserInterface/Environment/MDL_DISP/Traffic/Fellow_Movement/CurrentSegment[]1 ==
  In1 : Inport
  Out1 : Outport
  wires:
  In1/1 -> Out1/1

== system ASM_Traffic_V2X_Complete_Model_2/MDLUserInterface/Environment/MDL_DISP/Traffic/Fellow_Movement/CurrentSegment[]2 ==
  In1 : Inport
  Out1 : Outport
  wires:
  In1/1 -> Out1/1

== system ASM_Traffic_V2X_Complete_Model_2/MDLUserInterface/Environment/MDL_DISP/Traffic/Fellow_Movement/CurrentSequence[] ==
  In1 : Inport
  Out1 : Outport
  wires:
  In1/1 -> Out1/1

== system ASM_Traffic_V2X_Complete_Model_2/MDLUserInterface/Environment/MDL_DISP/Traffic/Fellow_Movement/CurrentSequence[]1 ==
  In1 : Inport
  Out1 : Outport
  wires:
  In1/1 -> Out1/1

== system ASM_Traffic_V2X_Complete_Model_2/MDLUserInterface/Environment/MDL_DISP/Traffic/Fellow_Movement/CurrentSequence[]2 ==
  In1 : Inport
  Out1 : Outport
  wires:
  In1/1 -> Out1/1

== system ASM_Traffic_V2X_Complete_Model_2/MDLUserInterface/Environment/MDL_DISP/Traffic/Fellow_Movement/FlagFellowUsed[0|1] ==
  In1 : Inport
  Out1 : Outport
  wires:
  In1/1 -> Out1/1

== system ASM_Traffic_V2X_Complete_Model_2/MDLUserInterface/Environment/MDL_DISP/Traffic/Fellow_Movement/FlagFellowUsed[0|1]1 ==
  In1 : Inport
  Out1 : Outport
  wires:
  In1/1 -> Out1/1

== system ASM_Traffic_V2X_Complete_Model_2/MDLUserInterface/Environment/MDL_DISP/Traffic/Fellow_Movement/FlagFellowUsed[0|1]2 ==
  In1 : Inport
  Out1 : Outport
  wires:
  In1/1 -> Out1/1

== system ASM_Traffic_V2X_Complete_Model_2/MDLUserInterface/Environment/MDL_DISP/Traffic/Fellow_Movement/GetFellowDataByIndex_1 ==
  SelectFellowDataByIndex : Inport
  TrafficBus : Inport  Port=2
  Saturation : Saturate  UpperLimit=MDL.Traffic.MaxNumFellows.v  LowerLimit=1
  SwitchFellowMovementData : Subsystem
  SwitchInfoData : Subsystem
  CurrentSequence[] : Outport
  CurrentSegment[] : Outport  Port=2
  t_local[s] : Outport  Port=3
  FlagFellowUsed[0|1] : Outport  Port=4
  s_Fellow[m] : Outport  Port=5
  d_Total_Fellow[m] : Outport  Port=6
  v_Fellow[km|h] : Outport  Port=7
  wires:
  Saturation/1 -> SwitchInfoData/2(Switch), SwitchFellowMovementData/2(Switch)
  SwitchInfoData/3(t_local[s]) -> t_local[s]/1
  SwitchFellowMovementData/1("Flag_Fellow_Used[0|1] ") -> FlagFellowUsed[0|1]/1
  SwitchFellowMovementData/4("v_Fellow[km|h] ") -> v_Fellow[km|h]/1
  SelectFellowDataByIndex/1 -> Saturation/1
  TrafficBus/1 -> SwitchInfoData/1(TrafficBus), SwitchFellowMovementData/1(TrafficBus)
  SwitchFellowMovementData/2("s_Fellow[m] ") -> s_Fellow[m]/1
  SwitchFellowMovementData/3("d_Total_Fellow[m] ") -> d_Total_Fellow[m]/1
  SwitchInfoData/2(CurrentSegment[]) -> CurrentSegment[]/1
  SwitchInfoData/1(CurrentSequence[]) -> CurrentSequence[]/1

== system ASM_Traffic_V2X_Complete_Model_2/MDLUserInterface/Environment/MDL_DISP/Traffic/Fellow_Movement/GetFellowDataByIndex_2 ==
  SelectFellowDataByIndex : Inport
  TrafficBus : Inport  Port=2
  Saturation : Saturate  UpperLimit=MDL.Traffic.MaxNumFellows.v  LowerLimit=1
  SwitchFellowMovementData : Subsystem
  SwitchInfoData : Subsystem
  CurrentSequence[] : Outport
  CurrentSegment[] : Outport  Port=2
  t_local[s] : Outport  Port=3
  FlagFellowUsed[0|1] : Outport  Port=4
  s_Fellow[m] : Outport  Port=5
  d_Total_Fellow[m] : Outport  Port=6
  v_Fellow[km|h] : Outport  Port=7
  wires:
  SwitchInfoData/1(CurrentSequence[]) -> CurrentSequence[]/1
  SwitchInfoData/2(CurrentSegment[]) -> CurrentSegment[]/1
  SwitchFellowMovementData/3("d_Total_Fellow[m] ") -> d_Total_Fellow[m]/1
  SwitchFellowMovementData/2("s_Fellow[m] ") -> s_Fellow[m]/1
  TrafficBus/1 -> SwitchFellowMovementData/1(TrafficBus), SwitchInfoData/1(TrafficBus)
  SelectFellowDataByIndex/1 -> Saturation/1
  SwitchFellowMovementData/4("v_Fellow[km|h] ") -> v_Fellow[km|h]/1
  SwitchFellowMovementData/1("Flag_Fellow_Used[0|1] ") -> FlagFellowUsed[0|1]/1
  SwitchInfoData/3(t_local[s]) -> t_local[s]/1
  Saturation/1 -> SwitchFellowMovementData/2(Switch), SwitchInfoData/2(Switch)

== system ASM_Traffic_V2X_Complete_Model_2/MDLUserInterface/Environment/MDL_DISP/Traffic/Fellow_Movement/GetFellowDataByIndex_3 ==
  SelectFellowDataByIndex : Inport
  TrafficBus : Inport  Port=2
  Saturation : Saturate  UpperLimit=MDL.Traffic.MaxNumFellows.v  LowerLimit=1
  SwitchFellowMovementData : Subsystem
  SwitchInfoData : Subsystem
  CurrentSequence[] : Outport
  CurrentSegment[] : Outport  Port=2
  t_local[s] : Outport  Port=3
  FlagFellowUsed[0|1] : Outport  Port=4
  s_Fellow[m] : Outport  Port=5
  d_Total_Fellow[m] : Outport  Port=6
  v_Fellow[km|h] : Outport  Port=7
  wires:
  Saturation/1 -> SwitchInfoData/2(Switch), SwitchFellowMovementData/2(Switch)
  SwitchInfoData/3(t_local[s]) -> t_local[s]/1
  SwitchFellowMovementData/1("Flag_Fellow_Used[0|1] ") -> FlagFellowUsed[0|1]/1
  SwitchFellowMovementData/4("v_Fellow[km|h] ") -> v_Fellow[km|h]/1
  SelectFellowDataByIndex/1 -> Saturation/1
  TrafficBus/1 -> SwitchInfoData/1(TrafficBus), SwitchFellowMovementData/1(TrafficBus)
  SwitchFellowMovementData/2("s_Fellow[m] ") -> s_Fellow[m]/1
  SwitchFellowMovementData/3("d_Total_Fellow[m] ") -> d_Total_Fellow[m]/1
  SwitchInfoData/2(CurrentSegment[]) -> CurrentSegment[]/1
  SwitchInfoData/1(CurrentSequence[]) -> CurrentSequence[]/1

== system ASM_Traffic_V2X_Complete_Model_2/MDLUserInterface/Environment/MDL_DISP/Traffic/Fellow_Movement/d_Total_Fellow[m] ==
  In1 : Inport
  Out1 : Outport
  wires:
  In1/1 -> Out1/1

== system ASM_Traffic_V2X_Complete_Model_2/MDLUserInterface/Environment/MDL_DISP/Traffic/Fellow_Movement/d_Total_Fellow[m]1 ==
  In1 : Inport
  Out1 : Outport
  wires:
  In1/1 -> Out1/1

== system ASM_Traffic_V2X_Complete_Model_2/MDLUserInterface/Environment/MDL_DISP/Traffic/Fellow_Movement/d_Total_Fellow[m]2 ==
  In1 : Inport
  Out1 : Outport
  wires:
  In1/1 -> Out1/1

== system ASM_Traffic_V2X_Complete_Model_2/MDLUserInterface/Environment/MDL_DISP/Traffic/Fellow_Movement/s_Fellow[m] ==
  In1 : Inport
  Out1 : Outport
  wires:
  In1/1 -> Out1/1

== system ASM_Traffic_V2X_Complete_Model_2/MDLUserInterface/Environment/MDL_DISP/Traffic/Fellow_Movement/s_Fellow[m]1 ==
  In1 : Inport
  Out1 : Outport
  wires:
  In1/1 -> Out1/1

== system ASM_Traffic_V2X_Complete_Model_2/MDLUserInterface/Environment/MDL_DISP/Traffic/Fellow_Movement/s_Fellow[m]2 ==
  In1 : Inport
  Out1 : Outport
  wires:
  In1/1 -> Out1/1

== system ASM_Traffic_V2X_Complete_Model_2/MDLUserInterface/Environment/MDL_DISP/Traffic/Fellow_Movement/t_local[s] ==
  In1 : Inport
  Out1 : Outport
  wires:
  In1/1 -> Out1/1

== system ASM_Traffic_V2X_Complete_Model_2/MDLUserInterface/Environment/MDL_DISP/Traffic/Fellow_Movement/t_local[s]1 ==
  In1 : Inport
  Out1 : Outport
  wires:
  In1/1 -> Out1/1

== system ASM_Traffic_V2X_Complete_Model_2/MDLUserInterface/Environment/MDL_DISP/Traffic/Fellow_Movement/t_local[s]2 ==
  In1 : Inport
  Out1 : Outport
  wires:
  In1/1 -> Out1/1

== system ASM_Traffic_V2X_Complete_Model_2/MDLUserInterface/Environment/MDL_DISP/Traffic/Fellow_Movement/v_Fellow[km|h] ==
  In1 : Inport
  Out1 : Outport
  wires:
  In1/1 -> Out1/1

== system ASM_Traffic_V2X_Complete_Model_2/MDLUserInterface/Environment/MDL_DISP/Traffic/Fellow_Movement/v_Fellow[km|h]1 ==
  In1 : Inport
  Out1 : Outport
  wires:
  In1/1 -> Out1/1

== system ASM_Traffic_V2X_Complete_Model_2/MDLUserInterface/Environment/MDL_DISP/Traffic/Fellow_Movement/v_Fellow[km|h]2 ==
  In1 : Inport
  Out1 : Outport
  wires:
  In1/1 -> Out1/1

== system ASM_Traffic_V2X_Complete_Model_2/MDLUserInterface/Environment/MDL_DISP/Traffic/Line_Sensor/Data_Valid[0|1|2] ==
  In1 : Inport
  Out1 : Outport
  wires:
  In1/1 -> Out1/1

== system ASM_Traffic_V2X_Complete_Model_2/MDLUserInterface/Environment/MDL_DISP/Traffic/Line_Sensor/Num_Pnts_Detected_Junction_Borders[] ==
  In1 : Inport
  Out1 : Outport
  wires:
  In1/1 -> Out1/1

== system ASM_Traffic_V2X_Complete_Model_2/MDLUserInterface/Environment/MDL_DISP/Traffic/Line_Sensor/Num_Pnts_Detected_Junction_Shape_ContObj[] ==
  In1 : Inport
  Out1 : Outport
  wires:
  In1/1 -> Out1/1

== system ASM_Traffic_V2X_Complete_Model_2/MDLUserInterface/Environment/MDL_DISP/Traffic/Line_Sensor/Num_Pnts_Detected_Junction_Shape_Lines[] ==
  In1 : Inport
  Out1 : Outport
  wires:
  In1/1 -> Out1/1

== system ASM_Traffic_V2X_Complete_Model_2/MDLUserInterface/Environment/MDL_DISP/Traffic/Line_Sensor/Num_Pnts_Detected_Road_Lanes[] ==
  In1 : Inport
  Out1 : Outport
  wires:
  In1/1 -> Out1/1

== system ASM_Traffic_V2X_Complete_Model_2/MDLUserInterface/Environment/MDL_DISP/Traffic/Line_Sensor/Num_Pnts_Detected_Road_Shape_ContObj[] ==
  In1 : Inport
  Out1 : Outport
  wires:
  In1/1 -> Out1/1

== system ASM_Traffic_V2X_Complete_Model_2/MDLUserInterface/Environment/MDL_DISP/Traffic/Line_Sensor/Num_Pnts_Detected_Road_Shape_Lines[] ==
  In1 : Inport
  Out1 : Outport
  wires:
  In1/1 -> Out1/1
